simulink subsystem "throttle"  (R2020b)
settings: Solver=VariableStepAuto  StartTime=0.0  StopTime=10.0  RelTol=1e-3
undefined symbols (not defined in the file): Cs, J, Kd, Ks, theta_eq
settings Model: Creator=bneiswan  LastModifiedBy=bneiswan

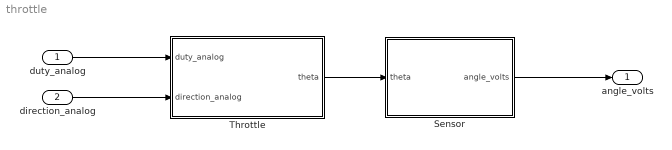
== system throttle ==
  duty_analog : Inport  OutDataTypeStr=double  PortDimensions=1  SampleTime=0
  direction_analog : Inport  Port=2  OutDataTypeStr=double  PortDimensions=1  SampleTime=0
  Sensor : Subsystem
  Throttle : Subsystem
  angle_volts : Outport  OutDataTypeStr=double  PortDimensions=1  SampleTime=0  VectorParamsAs1DForOutWhenUnconnected=off
  wires:
  duty_analog/1 -> Throttle/1(duty_analog)
  direction_analog/1 -> Throttle/2(direction_analog)
  Throttle/1(theta) -> Sensor/1(theta)
  Sensor/1(angle_volts) -> angle_volts/1

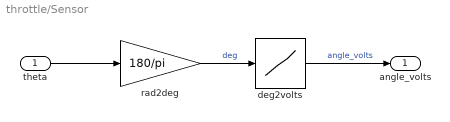
== system throttle/Sensor ==
  theta : Inport
  deg2volts : Lookup  InputValues=[0 90]  Table=[0.5 4.5]  LookUpMeth=Interpolation-Use End Values
  rad2deg : Gain  Gain=180/pi  SaturateOnIntegerOverflow=on  OutDataTypeStr=Inherit: Same as input  ParamDataTypeStr=Inherit: Same as input
  angle_volts : Outport  VectorParamsAs1DForOutWhenUnconnected=off
  wires:
  rad2deg/1 -> deg2volts/1  "deg"
  deg2volts/1 -> angle_volts/1  "angle_volts"
  theta/1 -> rad2deg/1

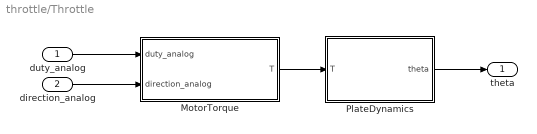
== system throttle/Throttle ==
  duty_analog : Inport
  direction_analog : Inport  Port=2
  MotorTorque : Subsystem
  PlateDynamics : Subsystem
  theta : Outport  VectorParamsAs1DForOutWhenUnconnected=off
  wires:
  PlateDynamics/1(theta) -> theta/1
  direction_analog/1 -> MotorTorque/2(direction_analog)
  duty_analog/1 -> MotorTorque/1(duty_analog)
  MotorTorque/1(T) -> PlateDynamics/1(T)

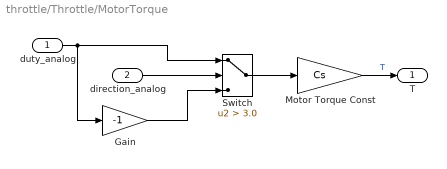
== system throttle/Throttle/MotorTorque ==
  duty_analog : Inport
  direction_analog : Inport  Port=2
  Gain : Gain  Gain=-1  SaturateOnIntegerOverflow=on  OutDataTypeStr=Inherit: Same as input  ParamDataTypeStr=Inherit: Same as input
  Motor Torque Const : Gain  Gain=Cs  SaturateOnIntegerOverflow=on  OutDataTypeStr=Inherit: Same as input  ParamDataTypeStr=Inherit: Same as input
  Switch : Switch  Criteria=u2 > Threshold  Threshold=3.0
  T : Outport  VectorParamsAs1DForOutWhenUnconnected=off
  wires:
  Motor Torque Const/1 -> T/1  "T"
  Gain/1 -> Switch/3
  duty_analog/1 -> Gain/1, Switch/1
  direction_analog/1 -> Switch/2
  Switch/1 -> Motor Torque Const/1

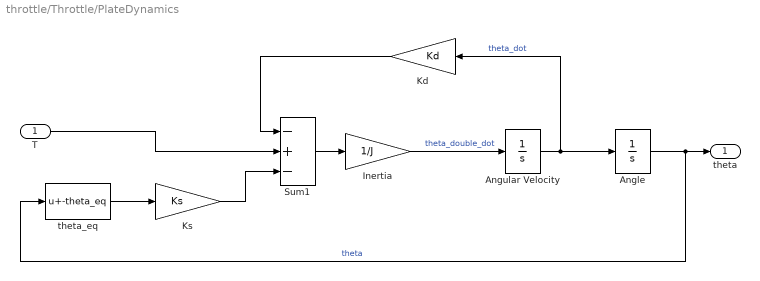
== system throttle/Throttle/PlateDynamics ==
  T : Inport
  Angle : Integrator  InitialCondition=theta_eq  LimitOutput=on  UpperSaturationLimit=pi/2  LowerSaturationLimit=0
      settings: AttributesFormatString=Initial condition: %<InitialCondition>\n%<LowerSaturationLimit> <= theta <= %<UpperSaturationLimit>
  Angular Velocity : Integrator
      settings: AttributesFormatString=Initial condition: %<InitialCondition>
  Inertia : Gain  Gain=1/J  SaturateOnIntegerOverflow=on  OutDataTypeStr=Inherit: Same as input  ParamDataTypeStr=Inherit: Same as input
  Kd : Gain  Gain=Kd  SaturateOnIntegerOverflow=on  OutDataTypeStr=Inherit: Same as input  ParamDataTypeStr=Inherit: Same as input
  Ks : Gain  Gain=Ks  SaturateOnIntegerOverflow=on  OutDataTypeStr=Inherit: Same as input  ParamDataTypeStr=Inherit: Same as input
  Sum1 : Sum  Inputs=-+-  SaturateOnIntegerOverflow=on
  theta_eq : Bias  Bias=-theta_eq
  theta : Outport  VectorParamsAs1DForOutWhenUnconnected=off
  wires:
  T/1 -> Sum1/2
  Ks/1 -> Sum1/3
  Kd/1 -> Sum1/1
  Sum1/1 -> Inertia/1
  Inertia/1 -> Angular Velocity/1  "theta_double_dot"
  Angular Velocity/1 -> Kd/1, Angle/1  "theta_dot"
  Angle/1 -> theta_eq/1, theta/1  "theta"
  theta_eq/1 -> Ks/1
